simulink model "P7"  (R2020b)
settings: Solver=VariableStepAuto  StartTime=0.0  StopTime=40  RelTol=1e-3
settings Model: Creator=abdullah  LastModifiedBy=abdullah

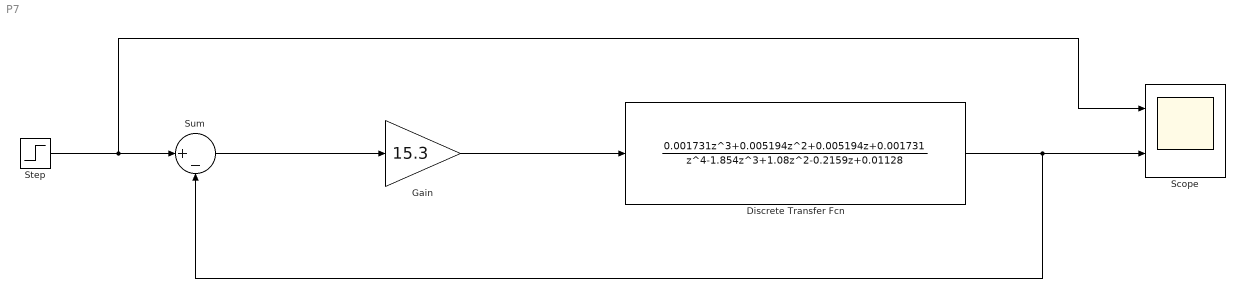
== system P7 ==
  Discrete Transfer Fcn : DiscreteTransferFcn  Numerator=[0.001731 0.005194 0.005194 0.001731]  Denominator=[1 -1.854 1.08 -0.2159 0.01128]  SampleTime=0.5
  Gain : Gain  Gain=15.3
  Scope : Scope  NumInputPorts=2
  Step : Step  SampleTime=0
  Sum : Sum  Inputs=|+-
  wires:
  Sum/1 -> Gain/1
  Gain/1 -> Discrete Transfer Fcn/1
  Step/1 -> Scope/1, Sum/1
  Discrete Transfer Fcn/1 -> Scope/2, Sum/2
